simulink model "rede_PLL_Pctedobro"  (Simulink 7.4)
settings: Solver=ode3  StartTime=0.0  StopTime=3  FixedStep=1e-3  MaxStep=1e-3  RelTol=1e-3
libraries: powerlib_extras x3, simulink_need_slupdate x2
settings Model: Creator=Batlab  LastModifiedBy=Batlab
settings OptimizationCC: InitFltsAndDblsToZero=on
settings DebuggingCC: SaveWithParameterizedLinksMsg=none
settings GRTTargetCC: TargetFcnLib=ansi_tfl_tmw.mat

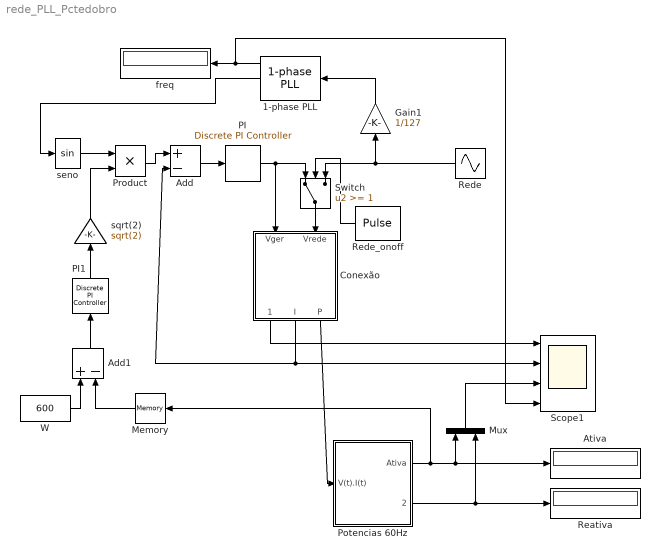
== system rede_PLL_Pctedobro ==
  1-phase PLL : powerlib_extras/Control  Blocks/1-phase PLL  DialogController=POWERSYS.PowerSysDialog  SystemSampleTime=-1  Par_Init=[0 60]  ParK=[ 180 3200 1 ]  AGC=off
  Add : Sum  Inputs=+-  OutDataType=sfix(16)  OutScaling=2^-10
  Add1 : Sum  Inputs=+-  OutDataType=sfix(16)  OutScaling=2^-10
  Ativa : Display
  Conexão : Subsystem
  Gain1 : Gain  Gain=1/127  ParameterDataType=sfix(16)  ParameterScaling=2^0  OutDataType=sfix(16)  OutScaling=2^0
  Memory : Memory
  Mux : Mux  Inputs=2
  PI : powerlib_extras/Discrete  Control Blocks/Discrete PI Controller  DialogController=POWERSYS.PowerSysDialog  SystemSampleTime=-1  Kp=10  Ki=20  Par_Limits=[1e3 -1e3]  Init=0  Ts=1e-3
  PI1 : powerlib_extras/Discrete  Control Blocks/Discrete PI Controller  DialogController=POWERSYS.PowerSysDialog  SystemSampleTime=-1  Kp=0.01  Ki=0.05  Par_Limits=[40 0]  Init=10  Ts=1e-3
  Potencias 60Hz : Subsystem
  Product : Product  OutDataType=sfix(16)  OutScaling=2^0  RndMeth=Zero
  Reativa : Display
  Rede : Sin  Amplitude=127*sqrt(2)  Bias=0  Frequency=60*2*pi  Phase=0  Samples=10  SampleTime=0  Offset=0
  Rede_onoff : DiscretePulseGenerator  PulseType=Time based  Amplitude=2  Period=2  PulseWidth=50  PhaseDelay=-1  SampleTime=1
  Scope1 : Scope  NumInputPorts=4
      settings: TimeRange=3  YMin=-200~-40~-2000~-5  YMax=200~20~4000~5  SaveName=dados
  Switch : Switch  Threshold=1
  W : Constant  Value=600  OutDataType=sfix(16)  OutScaling=2^0
  freq : Display
  seno : Trigonometry
  sqrt(2) : Gain  Gain=sqrt(2)  ParameterDataType=sfix(16)  ParameterScaling=2^0  OutDataType=sfix(16)  OutScaling=2^0
  wires:
  Conexão/1(Tensões) -> Scope1/1
  Conexão/3(P) -> Potencias 60Hz/1(V(t).I(t))
  Potencias 60Hz/2(Reativa) -> Reativa/1, Mux/2
  Potencias 60Hz/1(Ativa) -> Ativa/1, Mux/1, Memory/1
  Conexão/2(I) -> Add/2, Scope1/2
  Switch/1 -> Conexão/2(Vrede)
  Rede/1 -> Gain1/1, Switch/3
  1-phase PLL/1 -> freq/1, Scope1/4
  Gain1/1 -> 1-phase PLL/1
  seno/1 -> Product/1
  1-phase PLL/2 -> seno/1
  Rede_onoff/1 -> Switch/2
  Product/1 -> Add/1
  Add/1 -> PI/1
  PI/1 -> Switch/1, Conexão/1(Vger)
  Mux/1 -> Scope1/3
  sqrt(2)/1 -> Product/2
  Add1/1 -> PI1/1
  PI1/1 -> sqrt(2)/1
  W/1 -> Add1/1
  Memory/1 -> Add1/2

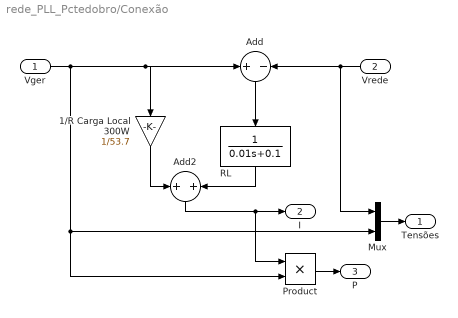
== system rede_PLL_Pctedobro/Conexão ==
  Vger : Inport  OutDataType=sfix(16)  OutScaling=2^0
  Vrede : Inport  Port=2  OutDataType=sfix(16)  OutScaling=2^0
  1/R Carga Local 300W : Gain  Gain=1/53.7  ParameterDataType=sfix(16)  ParameterScaling=2^0  OutDataType=sfix(16)  OutScaling=2^0
  Add : Sum  Inputs=+-  OutDataType=sfix(16)  OutScaling=2^-10
  Add2 : Sum  Inputs=2  OutDataType=sfix(16)  OutScaling=2^-10
  Mux : Mux  Inputs=2
  Product : Product  OutDataType=sfix(16)  OutScaling=2^0  RndMeth=Zero
  RL : TransferFcn  Denominator=[0.01 0.1]
  Tensões : Outport  OutDataType=sfix(16)  OutScaling=2^0
  I : Outport  Port=2  OutDataType=sfix(16)  OutScaling=2^0
  P : Outport  Port=3  OutDataType=sfix(16)  OutScaling=2^0
  wires:
  Vrede/1 -> Mux/1, Add/2
  Add/1 -> RL/1
  Vger/1 -> Product/2, Mux/2, Add/1, 1/R Carga Local 300W/1
  Mux/1 -> Tensões/1
  Product/1 -> P/1
  1/R Carga Local 300W/1 -> Add2/1
  Add2/1 -> I/1, Product/1
  RL/1 -> Add2/2

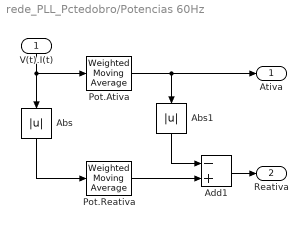
== system rede_PLL_Pctedobro/Potencias 60Hz ==
  V(t).I(t) : Inport  OutDataType=sfix(16)  OutScaling=2^0
  Abs : Abs
  Abs1 : Abs
  Add1 : Sum  Inputs=-+  OutDataType=sfix(16)  OutScaling=2^-10
  Pot.Ativa : simulink_need_slupdate/Weighted Moving Average  mgainval=[ones(1,16)]./16  vinit=0.0  samptime=-1  OutDataType=sfix(16)  OutScaling=2^-10  DoSatur=off  GainDataType=sfix( 16 )  MatRadixGroup=Best Precision: Matrix-wise  GainScaling=2^-10
  Pot.Reativa : simulink_need_slupdate/Weighted Moving Average  mgainval=[ones(1,16)]./16  vinit=0.0  samptime=-1  OutDataType=sfix(16)  OutScaling=2^-10  DoSatur=off  GainDataType=sfix( 16 )  MatRadixGroup=Best Precision: Matrix-wise  GainScaling=2^-10
  Ativa : Outport  OutDataType=sfix(16)  OutScaling=2^0
  Reativa : Outport  Port=2  OutDataType=sfix(16)  OutScaling=2^0
  wires:
  Abs/1 -> Pot.Reativa/1
  Pot.Reativa/1 -> Add1/2
  Pot.Ativa/1 -> Abs1/1, Ativa/1
  Abs1/1 -> Add1/1
  V(t).I(t)/1 -> Abs/1, Pot.Ativa/1
  Add1/1 -> Reativa/1
